simulink model "atrias_boom_nmSt_kinSw_v2"  (R2015a)
settings: Solver=ode23t  StartTime=0.0  StopTime=t_end  FixedStep=0.001  MaxStep=1e-3  RelTol=1e-3
InitFcn:
  | addpath('../common/')
  | colors
StartFcn:
  | tic
StopFcn:
  | %stopscript
values from neighbouring files (symbols this model uses):
  dt_a_dTrunk_boom = 5    [main_1_nmSt_kinSw.m]    (also in main_2_nmSt_kinSw_v2.m; main_3_nmSt_kinSw_v3.m; main_4_nmSt_kinSw_v4.m)
  dt_fade_boomCtrl = 2    [main_1_nmSt_kinSw.m]    (also in main_2_nmSt_kinSw_v2.m; main_3_nmSt_kinSw_v3.m; main_4_nmSt_kinSw_v4.m)
  initial_boom_yaw = 15*pi/180    (= 0.261799387799)    [main_2_nmSt_kinSw_v2.m]    (also in main_3_nmSt_kinSw_v3.m; main_4_nmSt_kinSw_v4.m)
  kd_boom_roll_Ctrl = 0    [main_1_nmSt_kinSw - Copy.m]    (also in main_1_nmSt_kinSw.m; main_2_nmSt_kinSw_v2.m; main_3_nmSt_kinSw_v3.m; main_4_nmSt_kinSw_v4.m)
  kd_boom_yaw_Ctrl = 0.1*kp_boom_yaw_Ctrl    (= 100000000)    [main_1_nmSt_kinSw - Copy.m]    (also in main_1_nmSt_kinSw.m = 1000000000; main_2_nmSt_kinSw_v2.m = 10000000; main_3_nmSt_kinSw_v3.m = 10000000; main_4_nmSt_kinSw_v4.m = 10000000)
  kd_motor = 0.90*2*sqrt(3.75*kp_motor)    [main_1_nmSt_kinSw - Copy.m]
  kinSw_alpha_start = 100*pi/180    (= 1.74532925199)    [main_1_nmSt_kinSw - Copy.m]    (also in main_1_nmSt_kinSw.m = 1.91986217719; main_2_nmSt_kinSw_v2.m = 1.83259571459; main_3_nmSt_kinSw_v3.m = 1.83259571459; main_4_nmSt_kinSw_v4.m = 1.83259571459)
  kinSw_alpha_tgt = 80*pi/180    (= 1.3962634016)    [main_1_nmSt_kinSw - Copy.m]    (also in main_1_nmSt_kinSw.m = 1.2217304764; main_2_nmSt_kinSw_v2.m = 1.2217304764; main_3_nmSt_kinSw_v3.m = 1.2217304764; main_4_nmSt_kinSw_v4.m = 1.2217304764)
  kinSw_t_start = 1.5    [main_1_nmSt_kinSw - Copy.m]    (also in main_1_nmSt_kinSw.m; main_2_nmSt_kinSw_v2.m = 0.5; main_3_nmSt_kinSw_v3.m = 0.5; main_4_nmSt_kinSw_v4.m = 0.5)
  kp_boom_roll_Ctrl = 0    [main_1_nmSt_kinSw - Copy.m]    (also in main_1_nmSt_kinSw.m; main_2_nmSt_kinSw_v2.m; main_3_nmSt_kinSw_v3.m; main_4_nmSt_kinSw_v4.m)
  kp_boom_yaw_Ctrl = 1e9    (= 1000000000)    [main_1_nmSt_kinSw - Copy.m]    (also in main_1_nmSt_kinSw.m = 10000000000; main_2_nmSt_kinSw_v2.m = 100000000; main_3_nmSt_kinSw_v3.m = 100000000; main_4_nmSt_kinSw_v4.m = 100000000)
  kp_motor = 3000    [main_1_nmSt_kinSw - Copy.m]
  max_back_bar_angle = 262.4*pi/180    (= 4.57974395723)    [main_1_nmSt_kinSw - Copy.m]
  max_front_bar_angle = 194.8*pi/180    (= 3.39990138288)    [main_1_nmSt_kinSw - Copy.m]
  min_back_bar_angle = 165.0*pi/180    (= 2.87979326579)    [main_1_nmSt_kinSw - Copy.m]
  min_front_bar_angle = 98.0*pi/180    (= 1.71042266695)    [main_1_nmSt_kinSw - Copy.m]
  poser_LLegAlp = (initial_l_leg_angle -pi/2)*180/pi    (= 105)    [main_2_nmSt_kinSw_v2.m]    (also in main_3_nmSt_kinSw_v3.m; main_4_nmSt_kinSw_v4.m)
  poser_LLegLen = initial_l_leg_length    (= 0.88)    [main_2_nmSt_kinSw_v2.m]    (also in main_3_nmSt_kinSw_v3.m; main_4_nmSt_kinSw_v4.m)
  poser_RLegAlp = (initial_r_leg_angle -pi/2)*180/pi    (= 75)    [main_2_nmSt_kinSw_v2.m]    (also in main_3_nmSt_kinSw_v3.m; main_4_nmSt_kinSw_v4.m)
  poser_RLegLen = initial_r_leg_length    (= 0.9)    [main_2_nmSt_kinSw_v2.m]    (also in main_3_nmSt_kinSw_v3.m; main_4_nmSt_kinSw_v4.m)
  tEnd_boomCtrl = t_end    (= 20)    [main_1_nmSt_kinSw - Copy.m]    (also in main_1_nmSt_kinSw.m = 3; main_2_nmSt_kinSw_v2.m = 7.5; main_3_nmSt_kinSw_v3.m = 7.5; main_4_nmSt_kinSw_v4.m = 7.5)
  tStart_boomCtrl = 1    [main_1_nmSt_kinSw - Copy.m]    (also in main_1_nmSt_kinSw.m = 0; main_2_nmSt_kinSw_v2.m = 0.5; main_3_nmSt_kinSw_v3.m = 0.5; main_4_nmSt_kinSw_v4.m = 0.5)
  tune_kinSw_alpha_start = kinSw_alpha_start*180/pi    (= 105)    [main_2_nmSt_kinSw_v2.m]    (also in main_3_nmSt_kinSw_v3.m; main_4_nmSt_kinSw_v4.m)
  tune_kinSw_alpha_tgt = kinSw_alpha_tgt*180/pi    (= 70)    [main_2_nmSt_kinSw_v2.m]    (also in main_3_nmSt_kinSw_v3.m; main_4_nmSt_kinSw_v4.m)
  tune_kinSw_len_min = kinSw_lclr    (= 0.7)    [main_2_nmSt_kinSw_v2.m]    (also in main_3_nmSt_kinSw_v3.m = 0.6)
  tune_kinSw_len_tgt = kinSw_len_tgt    (= 0.9)    [main_2_nmSt_kinSw_v2.m]    (also in main_3_nmSt_kinSw_v3.m)
  tune_M1_G = St_FGain_VAS*FmaxVAS    [main_2_nmSt_kinSw_v2.m]    (also in main_3_nmSt_kinSw_v3.m; main_4_nmSt_kinSw_v4.m)
  tune_M3_0 = CtrlPar_theta0*180/pi    [main_2_nmSt_kinSw_v2.m]    (also in main_3_nmSt_kinSw_v3.m; main_4_nmSt_kinSw_v4.m)
  tune_M3_D = St_GainDTh_HFL    [main_2_nmSt_kinSw_v2.m]    (also in main_3_nmSt_kinSw_v3.m; main_4_nmSt_kinSw_v4.m)
  tune_M3_P = St_GainTh_HFL    [main_2_nmSt_kinSw_v2.m]    (also in main_3_nmSt_kinSw_v3.m; main_4_nmSt_kinSw_v4.m)
  v_dTrunk_boom = 1.3    [main_1_nmSt_kinSw.m]    (also in main_2_nmSt_kinSw_v2.m; main_3_nmSt_kinSw_v3.m; main_4_nmSt_kinSw_v4.m)
undefined symbols (not defined in the file or in its folder): A1_notch_f1, A2_notch_f1, A_lpf_dtau, A_lpf_velocity, ankle_stiffness, B1_lpf_dtau, B1_lpf_velocity, B1_notch_f1, B2_lpf_dtau, B2_lpf_velocity, B2_notch_f1, b_hmotor, b_leg_spring, b_rotor, base_color_d, boom_color_d, boom_mount_to_center_diagonal, breakaway_friction, c_jointstop, contactThr, coulomb_friction, d_com, delta_phi_max, delta_phi_max_buffer, delta_phi_max_dropoff, delta_phi_min, fblink_color_d, floor_color_d, FmaxBFSH, FmaxGLU, FmaxHAM, FmaxHFL, FmaxRF, FmaxVAS, foot_color_d, FPCtrlPar, friction_linear_zone, g, gain_nodes_sea_torque, HIP_MTR_MAX_CONT_TORQUE, HIP_MTR_MAX_TORQUE, hshaft_color_d, initial_boom_pitch, initial_boom_roll, initial_hip_roll, initial_winch_angle, j_motor, k_gn, k_gt, k_leg_spring, K_notch_f1, k_phi, k_sea, Kb_leg, kd_lateral, kd_shin_max, kd_shin_min, kd_splay_max, kd_splay_min, kd_thigh_max ... (+187)
libraries: sm_lib x210, nesl_utility x140, simulink x65, simulink_extras x31, fl_lib x16, mblibv1 x2, commnoisgen2 x1
(part 4 of 16)

== system atrias_boom_nmSt_kinSw_v2/Mechanical System Layer/Right Hip Roll Joint ==
  note: Hip Roll Mechanics
  Hip Motor [Nm] : Inport
  1 / Gear Ratio : Gain  Gain=1/N_h
  Common Gear : sm_lib/Gears and Couplings/Gears/Common Gear Constraint  GearType=External  SpecificationType=PitchCircleRadii  CenterDistance=20.0  CenterDistanceUnits=cm  GearRatio=1.0  BaseGearRadius=r_hip_gearhead  BaseGearRadiusUnits=m  FollGearRadius=r_hip_shaft  FollGearRadiusUnits=m  AssemblyGearRotation=Free  BlockFunction=simmechanics.library.gears_couplings_drives.gears.common_gear
  Constant : Constant  Value=pi
  Damping : Gain  Gain=b_hmotor
  Hip Motor Frame : sm_lib/Frames and Transforms/Rigid Transform  TranslationMethod=Cartesian  TranslationLengthUnit=m  TranslationStandardAxis=+Z  TranslationStandardOffset=0  TranslationCartesianOffset=[0 r_hip_gearhead+r_hip_shaft 0]  TranslationROffset=0  TranslationROffsetUnits=m  TranslationZOffset=0  TranslationZOffsetUnits=m  TranslationThetaOffset=0  TranslationThetaOffsetUnits=deg  RotationMethod=None  RotationAngleUnits=deg  RotationStandardAxis=-Z  RotationAngle=180  RotationArbitraryAxis=[0 0 1]  FollAlignAxisA=-Z  BaseAlignAxisA=+Z  FollAlignAxisB=+Y  BaseAlignAxisB=+Y  RotationMatrix=[1 0 0; 0 1 0; 0 0 1]  BlockFunction=simmechanics.library.frames_transforms.rigid_transform
  Hip Roll Frame : sm_lib/Frames and Transforms/Rigid Transform  TranslationMethod=None  TranslationLengthUnit=m  TranslationStandardAxis=+Z  TranslationStandardOffset=0  TranslationCartesianOffset=[0 0 0]  TranslationROffset=0  TranslationROffsetUnits=m  TranslationZOffset=0  TranslationZOffsetUnits=m  TranslationThetaOffset=0  TranslationThetaOffsetUnits=deg  RotationMethod=AlignedAxes  RotationAngleUnits=deg  RotationStandardAxis=-Z  RotationAngle=180  RotationArbitraryAxis=[0 0 1]  FollAlignAxisA=+X  BaseAlignAxisA=+Z  FollAlignAxisB=+Y  BaseAlignAxisB=+Y  RotationMatrix=[1 0 0; 0 1 0; 0 0 1]  BlockFunction=simmechanics.library.frames_transforms.rigid_transform
  Hip Roll Joint : sm_lib/Joints/Revolute Joint  SenseConstraintForce=off  SenseConstraintForceX=off  SenseConstraintForceY=off  SenseConstraintForceZ=off  SenseConstraintTorque=off  SenseConstraintTorqueX=off  SenseConstraintTorqueY=off  SenseConstraintTorqueZ=off  SenseTotalForce=off  SenseTotalForceX=off  SenseTotalForceY=off  SenseTotalForceZ=off  SenseTotalTorque=off  SenseTotalTorqueX=off  SenseTotalTorqueY=off  SenseTotalTorqueZ=off  CompositeWrenchDir=FollowerOnBase  CompositeWrenchFrame=BaseFrame  EquilibriumPosition=0  EquilibriumPositionUnits=deg  SpringStiffness=0  SpringStiffnessUnits=N*m/deg  DampingCoefficient=0  DampingCoefficientUnits=N*m/(deg/s)  TorqueActuationMode=InputTorque  MotionActuationMode=ComputedMotion  SensePosition=on  SenseVelocity=on  SenseAcceleration=off  SenseTorqueForce=off  PositionTargetSpecify=on  PositionTargetPriority=High  PositionTargetValue=initial_hip_roll  PositionTargetValueUnits=rad  VelocityTargetSpecify=off  VelocityTargetPriority=High  VelocityTargetValue=0  VelocityTargetValueUnits=deg/s  BlockFunction=simmechanics.library.joints.revolute_joint
  Leg Frame : sm_lib/Frames and Transforms/Rigid Transform  TranslationMethod=None  TranslationLengthUnit=m  TranslationStandardAxis=+Z  TranslationStandardOffset=0  TranslationCartesianOffset=[0 0 0]  TranslationROffset=0  TranslationROffsetUnits=m  TranslationZOffset=0  TranslationZOffsetUnits=m  TranslationThetaOffset=0  TranslationThetaOffsetUnits=deg  RotationMethod=AlignedAxes  RotationAngleUnits=deg  RotationStandardAxis=-Z  RotationAngle=180  RotationArbitraryAxis=[0 0 1]  FollAlignAxisA=+Z  BaseAlignAxisA=+X  FollAlignAxisB=+Y  BaseAlignAxisB=+Y  RotationMatrix=[1 0 0; 0 1 0; 0 0 1]  BlockFunction=simmechanics.library.frames_transforms.rigid_transform
  "Mechanical Limits " : Subsystem
  Motor Efficiency : Gain  Gain=mu_hmotor
  Motor Joint : sm_lib/Joints/Revolute Joint  SenseConstraintForce=off  SenseConstraintForceX=off  SenseConstraintForceY=off  SenseConstraintForceZ=off  SenseConstraintTorque=off  SenseConstraintTorqueX=off  SenseConstraintTorqueY=off  SenseConstraintTorqueZ=off  SenseTotalForce=off  SenseTotalForceX=off  SenseTotalForceY=off  SenseTotalForceZ=off  SenseTotalTorque=off  SenseTotalTorqueX=off  SenseTotalTorqueY=off  SenseTotalTorqueZ=off  CompositeWrenchDir=FollowerOnBase  CompositeWrenchFrame=BaseFrame  EquilibriumPosition=0  EquilibriumPositionUnits=deg  SpringStiffness=0  SpringStiffnessUnits=N*m/deg  DampingCoefficient=0  DampingCoefficientUnits=N*m/(deg/s)  TorqueActuationMode=InputTorque  MotionActuationMode=ComputedMotion  SensePosition=off  SenseVelocity=on  SenseAcceleration=off  SenseTorqueForce=off  PositionTargetSpecify=off  PositionTargetPriority=Low  PositionTargetValue=30  PositionTargetValueUnits=deg  VelocityTargetSpecify=off  VelocityTargetPriority=High  VelocityTargetValue=0  VelocityTargetValueUnits=deg/s  BlockFunction=simmechanics.library.joints.revolute_joint
  PS-Simulink Converter : nesl_utility/PS-Simulink Converter  PhysicalDomain=network_engine_domain  SubClassName=ps_output  LeftPortType=input  RightPortType=output  PseudoPeriodic=off  Frequencies=[]  Unit=1  AffineConversion=off
  PS-Simulink Converter1 : nesl_utility/PS-Simulink Converter  PhysicalDomain=network_engine_domain  SubClassName=ps_output  LeftPortType=input  RightPortType=output  PseudoPeriodic=off  Frequencies=[]  Unit=1  AffineConversion=off
  PS-Simulink Converter3 : nesl_utility/PS-Simulink Converter  PhysicalDomain=network_engine_domain  SubClassName=ps_output  LeftPortType=input  RightPortType=output  PseudoPeriodic=off  Frequencies=[]  Unit=1  AffineConversion=off
  Rotor : sm_lib/Body Elements/Solid  InertiaType=Custom  Mass=0  MassUnits=kg  CenterOfMass=[0 0 0]  CenterOfMassUnits=m  MomentsOfInertia=i_hrotor_moments  MomentsOfInertiaUnits=kg*m^2  ProductsOfInertia=[0 0 0]  ProductsOfInertiaUnits=kg*m^2  DensityBased=on  Density=1000  DensityUnits=kg/(m^3)  GraphicType=None  MarkerShape=Sphere  MarkerSize=10  MarkerSizeUnits=m  GraphicVisPropType=AdvancedVisualProperties  GraphicDiffuseColor=hshaft_color_d  GraphicSpecularColor=[0.5 0.5 0.5 1.0]  GraphicAmbientColor=[0.15 0.15 0.15 1.0]  GraphicEmissiveColor=[0.0 0.0 0.0 1.0]  GraphicShininess=10  GraphicOpacity=1.0  GeometryShape=Cylinder  RectangleSize=[1 1]  RectangleSizeUnits=m  BrickDimensions=[1 1 1]  BrickDimensionUnits=m  CylinderRadius=0.1  CylinderRadiusUnits=m  CylinderLength=0.1  CylinderLengthUnits=m  SphereRadius=1  SphereRadiusUnits=m  EllipsoidRadii=[1 1 1]  EllipsoidRadiiUnits=m  ExtrusionCrossSection=[1 1; -1 1; -1 -1; 1 -1]  ExtrusionCrossSectionUnits=m  ExtrusionLength=1  ExtrusionLengthUnits=m  PolygonNumSides=3  PolygonOuterRadius=1  PolygonOuterRadiusUnits=m  ExtGeomFileType=STL  ExtGeomFileUnits=m  RevolutionCrossSection=[1 1; 1 -1; 2 -1; 2 1]  RevolutionCrossSectionUnits=m  RevolutionExtent=Full  RevolutionAngle=180  RevolutionAngleUnits=deg  BlockFunction=simmechanics.library.body_elements.solid
  Simulink-PS Converter : nesl_utility/Simulink-PS Converter  PhysicalDomain=network_engine_domain  SubClassName=ps_input  LeftPortType=input  RightPortType=output  PseudoPeriodic=off  Frequencies=[]  NoiseDistribution=none  NoiseParameters=[]  Unit=1  AffineConversion=off  InputFiltering=off  SimscapeFilterOrder=1  InputFilterTimeConstant=0.001  UdotUserProvided=1
  Simulink-PS Converter1 : nesl_utility/Simulink-PS Converter  PhysicalDomain=network_engine_domain  SubClassName=ps_input  LeftPortType=input  RightPortType=output  PseudoPeriodic=off  Frequencies=[]  NoiseDistribution=none  NoiseParameters=[]  Unit=1  AffineConversion=off  InputFiltering=off  SimscapeFilterOrder=1  InputFilterTimeConstant=0.001  UdotUserProvided=1
  Sum : Sum  Inputs=|+-
  Sum1 : Sum  Inputs=++|
  Torque Limiter (outside) 1 : Saturate  UpperLimit=HIP_MTR_MAX_TORQUE  LowerLimit=-HIP_MTR_MAX_TORQUE  ZeroCross=off
      settings: AttributesFormatString=Hi: %<UpperLimit>\nLo: %<LowerLimit>
  Leg Hip Conn : PMIOPort  Port=1  Side=Right
  Torso Hip Conn : PMIOPort  Port=2  Side=Left
  Hip Roll [rad] : Outport
  wires:
  Motor Efficiency/1 -> Simulink-PS Converter1/1
  Sum/1 -> Motor Efficiency/1
  Damping/1 -> Sum/2
  PS-Simulink Converter3/1 -> Damping/1
  Constant/1 -> Sum1/2
  Hip Motor [Nm]/1 -> Torque Limiter (outside) 1/1
  1 / Gear Ratio/1 -> Sum/1
  PS-Simulink Converter1/1 -> "Mechanical Limits "/1(vphi)
  Sum1/1 -> "Mechanical Limits "/2(phi)
  PS-Simulink Converter/1 -> Hip Roll [rad]/1, Sum1/1
  "Mechanical Limits "/1(tau_reaction) -> Simulink-PS Converter/1
  Torque Limiter (outside) 1/1 -> 1 / Gear Ratio/1
  connections:
  Hip Roll Frame/RConn1 -- Hip Roll Joint/LConn1 -- Hip Motor Frame/LConn1
  Simulink-PS Converter/RConn1 -- Hip Roll Joint/LConn2
  PS-Simulink Converter/LConn1 -- Hip Roll Joint/RConn2
  PS-Simulink Converter1/LConn1 -- Hip Roll Joint/RConn3
  Hip Roll Frame/LConn1 -- Torso Hip Conn/RConn1
  Leg Frame/RConn1 -- Leg Hip Conn/RConn1
  Motor Joint/RConn2 -- PS-Simulink Converter3/LConn1
  Simulink-PS Converter1/RConn1 -- Motor Joint/LConn2
  Leg Frame/LConn1 -- Common Gear/RConn1 -- Hip Roll Joint/RConn1
  Hip Motor Frame/RConn1 -- Motor Joint/LConn1
  Rotor/RConn1 -- Common Gear/LConn1 -- Motor Joint/RConn1

== system atrias_boom_nmSt_kinSw_v2/Mechanical System Layer/Torso ==
  COM Sensor : Subsystem
  COM accelerations : Scope
      settings: TimeRange=3  YMin=-750  YMax=2750  SaveName=ScopeData27
  COM dx : Scope
      settings: TimeRange=4  YMin=2.65  YMax=3.5  SaveName=ScopeData24
  COM dy : Scope
      settings: TimeRange=4  YMin=-1.25  YMax=1.5  SaveName=ScopeData32
  COM y pos : Scope
      settings: TimeRange=3  YMin=0.825  YMax=1.025  SaveName=ScopeData23
  CS1 to CS2 : sm_lib/Frames and Transforms/Rigid Transform  TranslationMethod=Cartesian  TranslationLengthUnit=m  TranslationStandardAxis=+Z  TranslationStandardOffset=0  TranslationCartesianOffset=torso_12  TranslationROffset=0  TranslationROffsetUnits=m  TranslationZOffset=0  TranslationZOffsetUnits=m  TranslationThetaOffset=0  TranslationThetaOffsetUnits=deg  RotationMethod=None  RotationAngleUnits=deg  RotationStandardAxis=+Z  RotationAngle=0  RotationArbitraryAxis=[0 0 1]  FollAlignAxisA=+X  BaseAlignAxisA=+Y  FollAlignAxisB=+Y  BaseAlignAxisB=+Z  RotationMatrix=[1 0 0; 0 1 0; 0 0 1]  BlockFunction=simmechanics.library.frames_transforms.rigid_transform
  Frame Data : Subsystem
  Hip Point to COM : sm_lib/Frames and Transforms/Rigid Transform  TranslationMethod=Cartesian  TranslationLengthUnit=m  TranslationStandardAxis=+Z  TranslationStandardOffset=0  TranslationCartesianOffset=[0 d_com 0]  TranslationROffset=0  TranslationROffsetUnits=m  TranslationZOffset=0  TranslationZOffsetUnits=m  TranslationThetaOffset=0  TranslationThetaOffsetUnits=deg  RotationMethod=None  RotationAngleUnits=deg  RotationStandardAxis=+Z  RotationAngle=0  RotationArbitraryAxis=[0 0 1]  FollAlignAxisA=+X  BaseAlignAxisA=+Y  FollAlignAxisB=+Y  BaseAlignAxisB=+Z  RotationMatrix=[1 0 0; 0 1 0; 0 0 1]  BlockFunction=simmechanics.library.frames_transforms.rigid_transform
  Mux : Mux  Inputs=2
  Solid : sm_lib/Body Elements/Solid  InertiaType=Custom  Mass=m_torso  MassUnits=kg  CenterOfMass=com_torso  CenterOfMassUnits=m  MomentsOfInertia=i_torso_moments  MomentsOfInertiaUnits=kg*m^2  ProductsOfInertia=i_torso_products  ProductsOfInertiaUnits=kg*m^2  DensityBased=on  Density=1000  DensityUnits=kg/(m^3)  GraphicType=FromGeometry  MarkerShape=Sphere  MarkerSize=10  MarkerSizeUnits=m  GraphicVisPropType=AdvancedVisualProperties  GraphicDiffuseColor=torso_color_d  GraphicSpecularColor=[0.5 0.5 0.5 1.0]  GraphicAmbientColor=[torso_color_d*0.5 1.0]  GraphicEmissiveColor=[0.0 0.0 0.0 1.0]  GraphicShininess=128  GraphicOpacity=1.0  GeometryShape=FromFile  RectangleSize=[1 1]  RectangleSizeUnits=m  BrickDimensions=[1 1 1]  BrickDimensionUnits=m  CylinderRadius=l_rad  CylinderRadiusUnits=m  CylinderLength=l_seg  CylinderLengthUnits=m  SphereRadius=1  SphereRadiusUnits=m  EllipsoidRadii=[1 1 1]  EllipsoidRadiiUnits=m  ExtrusionCrossSection=[1 1; -1 1; -1 -1; 1 -1]  ExtrusionCrossSectionUnits=m  ExtrusionLength=1  ExtrusionLengthUnits=m  PolygonNumSides=3  PolygonOuterRadius=1  PolygonOuterRadiusUnits=m  ExtGeomFileType=STL  ExtGeomFileName=../models/torso.STL  ExtGeomFileUnits=m  RevolutionCrossSection=[1 1; 1 -1; 2 -1; 2 1]  RevolutionCrossSectionUnits=m  RevolutionExtent=Full  RevolutionAngle=180  RevolutionAngleUnits=deg  BlockFunction=simmechanics.library.body_elements.solid
  Sum : Sum  Inputs=|++
  Total Energy : Scope
      settings: TimeRange=4  YMin=750  YMax=1025  SaveName=ScopeData22
  kinetic : Fcn  Expr=0.5*(u(1)^2+u(2)^2)*(m_total+m_boom/2)
  potential : Fcn  Expr=u*(m_total+m_boom/2)*g
  CS1 : PMIOPort  Port=1  Side=Right
  CS2 : PMIOPort  Port=2  Side=Left
  CS3 : PMIOPort  Port=3  Side=Left
  wires:
  COM Sensor/3(dx) -> Mux/1, COM dx/1
  COM Sensor/1(Acceleration) -> COM accelerations/1
  COM Sensor/4(dy) -> COM dy/1, Mux/2
  Mux/1 -> kinetic/1
  COM Sensor/2(y) -> COM y pos/1, potential/1
  kinetic/1 -> Sum/1
  potential/1 -> Sum/2
  Sum/1 -> Total Energy/1
  connections:
  CS1 to CS2/LConn1 -- Frame Data/LConn1 -- CS1/RConn1 -- Solid/RConn1
  CS3/RConn1 -- CS2/RConn1 -- Hip Point to COM/LConn1 -- CS1 to CS2/RConn1
  Hip Point to COM/RConn1 -- COM Sensor/LConn1

== system atrias_boom_nmSt_kinSw_v2/Mechanical System Layer/Winch ==
  note: Cable cannot push
  boom_roll_ctrl [Nm] : Inport
  Compare To Constant1 : simulink/Logic and Bit Operations/Compare To Constant  relop===  const=-1  OutDataTypeStr=boolean  ZeroCross=off
  Constant1 : Constant  Value=initial_winch_angle
  Constant2 : Constant  Value=0
  Desired Roll Velocity : Constant  Value=0
  Gain1 : Gain  Gain=kp_winch
  Gain3 : Gain  Gain=kd_winch
  PS-Simulink Converter : nesl_utility/PS-Simulink Converter  PhysicalDomain=network_engine_domain  SubClassName=ps_output  LeftPortType=input  RightPortType=output  PseudoPeriodic=off  Frequencies=[]  Unit=1  AffineConversion=off
  PS-Simulink Converter1 : nesl_utility/PS-Simulink Converter  PhysicalDomain=network_engine_domain  SubClassName=ps_output  LeftPortType=input  RightPortType=output  PseudoPeriodic=off  Frequencies=[]  Unit=1  AffineConversion=off
  Pitch Frame : sm_lib/Frames and Transforms/Rigid Transform  TranslationMethod=None  TranslationLengthUnit=m  TranslationStandardAxis=+Z  TranslationStandardOffset=0  TranslationCartesianOffset=[0 0 0]  TranslationROffset=0  TranslationROffsetUnits=m  TranslationZOffset=0  TranslationZOffsetUnits=m  TranslationThetaOffset=0  TranslationThetaOffsetUnits=deg  RotationMethod=AlignedAxes  RotationAngleUnits=rad  RotationStandardAxis=+Z  RotationAngle=0  RotationArbitraryAxis=[1 0 0]  FollAlignAxisA=-Z  BaseAlignAxisA=+X  FollAlignAxisB=+Y  BaseAlignAxisB=+Y  RotationMatrix=[1 0 0; 0 1 0; 0 0 1]  BlockFunction=simmechanics.library.frames_transforms.rigid_transform
  Roll Frame : sm_lib/Frames and Transforms/Rigid Transform  TranslationMethod=None  TranslationLengthUnit=m  TranslationStandardAxis=+Z  TranslationStandardOffset=0  TranslationCartesianOffset=[0 0 0]  TranslationROffset=0  TranslationROffsetUnits=m  TranslationZOffset=0  TranslationZOffsetUnits=m  TranslationThetaOffset=0  TranslationThetaOffsetUnits=deg  RotationMethod=AlignedAxes  RotationAngleUnits=rad  RotationStandardAxis=+Z  RotationAngle=0  RotationArbitraryAxis=[1 0 0]  FollAlignAxisA=+X  BaseAlignAxisA=-Z  FollAlignAxisB=+Y  BaseAlignAxisB=+Y  RotationMatrix=[1 0 0; 0 1 0; 0 0 1]  BlockFunction=simmechanics.library.frames_transforms.rigid_transform
  Roll Joint : sm_lib/Joints/Revolute Joint  SenseConstraintForce=off  SenseConstraintForceX=off  SenseConstraintForceY=off  SenseConstraintForceZ=off  SenseConstraintTorque=off  SenseConstraintTorqueX=off  SenseConstraintTorqueY=off  SenseConstraintTorqueZ=off  SenseTotalForce=off  SenseTotalForceX=off  SenseTotalForceY=off  SenseTotalForceZ=off  SenseTotalTorque=off  SenseTotalTorqueX=off  SenseTotalTorqueY=off  SenseTotalTorqueZ=off  CompositeWrenchDir=FollowerOnBase  CompositeWrenchFrame=BaseFrame  EquilibriumPosition=0  EquilibriumPositionUnits=deg  SpringStiffness=0  SpringStiffnessUnits=N*m/deg  DampingCoefficient=0  DampingCoefficientUnits=N*m/(deg/s)  TorqueActuationMode=InputTorque  MotionActuationMode=ComputedMotion  SensePosition=on  SenseVelocity=on  SenseAcceleration=off  SenseTorqueForce=off  PositionTargetSpecify=on  PositionTargetPriority=High  PositionTargetValue=initial_boom_roll  PositionTargetValueUnits=rad  VelocityTargetSpecify=off  VelocityTargetPriority=High  VelocityTargetValue=0  VelocityTargetValueUnits=deg/s  BlockFunction=simmechanics.library.joints.revolute_joint
  Sign1 : Signum  ZeroCross=off
  Simulink-PS Converter : nesl_utility/Simulink-PS Converter  PhysicalDomain=network_engine_domain  SubClassName=ps_input  LeftPortType=input  RightPortType=output  PseudoPeriodic=off  Frequencies=[]  NoiseDistribution=none  NoiseParameters=[]  Unit=1  AffineConversion=off  InputFiltering=off  SimscapeFilterOrder=1  InputFilterTimeConstant=0.001  UdotUserProvided=1
  Sum : Sum  Inputs=+-|
  Sum1 : Sum  Inputs=+|+
  Sum2 : Sum  Inputs=|++
  Sum3 : Sum  Inputs=+-|
  Switch : Switch  Threshold=1
  Boom : PMIOPort  Port=1  Side=Right
  Yaw Shaft : PMIOPort  Port=2  Side=Right
  Boom Roll [rad] : Outport
  wires:
  Sum/1 -> Gain1/1
  Sum1/1 -> Switch/3, Sign1/1
  Sign1/1 -> Compare To Constant1/1
  Constant2/1 -> Switch/1
  Compare To Constant1/1 -> Switch/2
  PS-Simulink Converter/1 -> Boom Roll [rad]/1, Sum/2
  PS-Simulink Converter1/1 -> Sum3/2
  Desired Roll Velocity/1 -> Sum3/1
  Sum3/1 -> Gain3/1
  Gain1/1 -> Sum1/1
  Gain3/1 -> Sum1/2
  Constant1/1 -> Sum/1
  Switch/1 -> Sum2/1
  Sum2/1 -> Simulink-PS Converter/1
  boom_roll_ctrl [Nm]/1 -> Sum2/2
  connections:
  Roll Frame/RConn1 -- Roll Joint/LConn1
  Roll Frame/LConn1 -- Yaw Shaft/RConn1
  Boom/RConn1 -- Pitch Frame/RConn1
  Pitch Frame/LConn1 -- Roll Joint/RConn1
  Roll Joint/LConn2 -- Simulink-PS Converter/RConn1
  PS-Simulink Converter/LConn1 -- Roll Joint/RConn2
  PS-Simulink Converter1/LConn1 -- Roll Joint/RConn3

== system atrias_boom_nmSt_kinSw_v2/Mechanical System Layer/Yaw Joint ==
  boom_yaw_ctrl [Nm] : Inport
  PS-Simulink Converter3 : nesl_utility/PS-Simulink Converter  PhysicalDomain=network_engine_domain  SubClassName=ps_output  LeftPortType=input  RightPortType=output  PseudoPeriodic=off  Frequencies=[]  Unit=1  AffineConversion=off
  Roll Frame : sm_lib/Frames and Transforms/Rigid Transform  TranslationMethod=None  TranslationLengthUnit=m  TranslationStandardAxis=+Z  TranslationStandardOffset=0  TranslationCartesianOffset=[0 0 0]  TranslationROffset=0  TranslationROffsetUnits=m  TranslationZOffset=0  TranslationZOffsetUnits=m  TranslationThetaOffset=0  TranslationThetaOffsetUnits=deg  RotationMethod=AlignedAxes  RotationAngleUnits=rad  RotationStandardAxis=+Z  RotationAngle=0  RotationArbitraryAxis=[1 0 0]  FollAlignAxisA=+Z  BaseAlignAxisA=+Y  FollAlignAxisB=+X  BaseAlignAxisB=+X  RotationMatrix=[1 0 0; 0 1 0; 0 0 1]  BlockFunction=simmechanics.library.frames_transforms.rigid_transform
  Simulink-PS Converter : nesl_utility/Simulink-PS Converter  PhysicalDomain=network_engine_domain  SubClassName=ps_input  LeftPortType=input  RightPortType=output  PseudoPeriodic=off  Frequencies=[]  NoiseDistribution=none  NoiseParameters=[]  Unit=1  AffineConversion=off  InputFiltering=off  SimscapeFilterOrder=1  InputFilterTimeConstant=0.001  UdotUserProvided=1
  Yaw Frame : sm_lib/Frames and Transforms/Rigid Transform  TranslationMethod=None  TranslationLengthUnit=m  TranslationStandardAxis=+Z  TranslationStandardOffset=0  TranslationCartesianOffset=[0 0 0]  TranslationROffset=0  TranslationROffsetUnits=m  TranslationZOffset=0  TranslationZOffsetUnits=m  TranslationThetaOffset=0  TranslationThetaOffsetUnits=deg  RotationMethod=AlignedAxes  RotationAngleUnits=rad  RotationStandardAxis=+Z  RotationAngle=0  RotationArbitraryAxis=[1 0 0]  FollAlignAxisA=+Y  BaseAlignAxisA=+Z  FollAlignAxisB=+X  BaseAlignAxisB=+X  RotationMatrix=[1 0 0; 0 1 0; 0 0 1]  BlockFunction=simmechanics.library.frames_transforms.rigid_transform
  Yaw Joint : sm_lib/Joints/Revolute Joint  SenseConstraintForce=off  SenseConstraintForceX=off  SenseConstraintForceY=off  SenseConstraintForceZ=off  SenseConstraintTorque=off  SenseConstraintTorqueX=off  SenseConstraintTorqueY=off  SenseConstraintTorqueZ=off  SenseTotalForce=off  SenseTotalForceX=off  SenseTotalForceY=off  SenseTotalForceZ=off  SenseTotalTorque=off  SenseTotalTorqueX=off  SenseTotalTorqueY=off  SenseTotalTorqueZ=off  CompositeWrenchDir=FollowerOnBase  CompositeWrenchFrame=BaseFrame  EquilibriumPosition=0  EquilibriumPositionUnits=deg  SpringStiffness=0  SpringStiffnessUnits=N*m/deg  DampingCoefficient=0  DampingCoefficientUnits=N*m/(deg/s)  TorqueActuationMode=InputTorque  MotionActuationMode=ComputedMotion  SensePosition=on  SenseVelocity=off  SenseAcceleration=off  SenseTorqueForce=off  PositionTargetSpecify=on  PositionTargetPriority=High  PositionTargetValue=initial_boom_yaw  PositionTargetValueUnits=rad  VelocityTargetSpecify=on  VelocityTargetPriority=High  VelocityTargetValue=initial_boom_yaw_velocity  VelocityTargetValueUnits=rad/s  BlockFunction=simmechanics.library.joints.revolute_joint
  Yaw Shaft : PMIOPort  Port=1  Side=Right
  Base : PMIOPort  Port=2  Side=Left
  Yaw [rad] : Outport
  wires:
  PS-Simulink Converter3/1 -> Yaw [rad]/1
  boom_yaw_ctrl [Nm]/1 -> Simulink-PS Converter/1
  connections:
  Yaw Frame/LConn1 -- Base/RConn1
  Yaw Joint/LConn1 -- Yaw Frame/RConn1
  Roll Frame/LConn1 -- Yaw Joint/RConn1
  Roll Frame/RConn1 -- Yaw Shaft/RConn1
  PS-Simulink Converter3/LConn1 -- Yaw Joint/RConn2
  Simulink-PS Converter/RConn1 -- Yaw Joint/LConn2

== system atrias_boom_nmSt_kinSw_v2/Mechanical System Layer/Yaw Shaft ==
  CS1 to CS2 : sm_lib/Frames and Transforms/Rigid Transform  TranslationMethod=Cartesian  TranslationLengthUnit=m  TranslationStandardAxis=+Z  TranslationStandardOffset=0  TranslationCartesianOffset=yshaft_12  TranslationROffset=0  TranslationROffsetUnits=m  TranslationZOffset=0  TranslationZOffsetUnits=m  TranslationThetaOffset=0  TranslationThetaOffsetUnits=deg  RotationMethod=None  RotationAngleUnits=deg  RotationStandardAxis=+Z  RotationAngle=0  RotationArbitraryAxis=[0 0 1]  FollAlignAxisA=+X  BaseAlignAxisA=+Y  FollAlignAxisB=+Y  BaseAlignAxisB=+Z  RotationMatrix=[1 0 0; 0 1 0; 0 0 1]  BlockFunction=simmechanics.library.frames_transforms.rigid_transform
  Frame Data : Subsystem
  Solid : sm_lib/Body Elements/Solid  InertiaType=Custom  Mass=m_yshaft  MassUnits=kg  CenterOfMass=com_yshaft  CenterOfMassUnits=m  MomentsOfInertia=i_yshaft_moments  MomentsOfInertiaUnits=kg*m^2  ProductsOfInertia=i_yshaft_products  ProductsOfInertiaUnits=kg*m^2  DensityBased=on  Density=1000  DensityUnits=kg/(m^3)  GraphicType=FromGeometry  MarkerShape=Sphere  MarkerSize=10  MarkerSizeUnits=m  GraphicVisPropType=AdvancedVisualProperties  GraphicDiffuseColor=yshaft_color_d  GraphicSpecularColor=[0.5 0.5 0.5 1.0]  GraphicAmbientColor=[yshaft_color_d*0.5 1.0]  GraphicEmissiveColor=[0.0 0.0 0.0 1.0]  GraphicShininess=128  GraphicOpacity=1.0  GeometryShape=FromFile  RectangleSize=[1 1]  RectangleSizeUnits=m  BrickDimensions=[1 1 1]  BrickDimensionUnits=m  CylinderRadius=l_rad  CylinderRadiusUnits=m  CylinderLength=l_seg  CylinderLengthUnits=m  SphereRadius=1  SphereRadiusUnits=m  EllipsoidRadii=[1 1 1]  EllipsoidRadiiUnits=m  ExtrusionCrossSection=[1 1; -1 1; -1 -1; 1 -1]  ExtrusionCrossSectionUnits=m  ExtrusionLength=1  ExtrusionLengthUnits=m  PolygonNumSides=3  PolygonOuterRadius=1  PolygonOuterRadiusUnits=m  ExtGeomFileType=STL  ExtGeomFileName=../models/boom_yaw.stl  ExtGeomFileUnits=m  RevolutionCrossSection=[1 1; 1 -1; 2 -1; 2 1]  RevolutionCrossSectionUnits=m  RevolutionExtent=Full  RevolutionAngle=180  RevolutionAngleUnits=deg  BlockFunction=simmechanics.library.body_elements.solid
  CS1 : PMIOPort  Port=1  Side=Left
  CS2 : PMIOPort  Port=2  Side=Right
  connections:
  CS2/RConn1 -- CS1 to CS2/RConn1
  CS1/RConn1 -- CS1 to CS2/LConn1 -- Solid/RConn1 -- Frame Data/LConn1

== system atrias_boom_nmSt_kinSw_v2/boom Ctrl/boom Ctrl ==
  Boom Roll [rad] : Inport
  Boom Yaw [rad] : Inport  Port=2
  Enable : EnablePort
  Constant1 : Constant  Value=initial_boom_yaw
  Constant2 : Constant  Value=l_boom+boom_mount_to_center_diagonal
  Constant3 : Constant  Value=initial_boom_roll
  Derivative : Derivative
  Derivative1 : Derivative
  Desired Roll Velocity1 : Constant  Value=0
  Desired Roll Velocity2 : Constant  Value=0
  Divide : Product  Inputs=*/
  Divide1 : Product
  Divide2 : Product
  Gain1 : Gain  Gain=kd_boom_roll_Ctrl
  Gain2 : Gain  Gain=kp_boom_roll_Ctrl
  Gain3 : Gain  Gain=kd_boom_yaw_Ctrl
  Gain4 : Gain  Gain=kp_boom_yaw_Ctrl
  Gain5 : Gain  Gain=180/pi
  Gain6 : Gain  Gain=180/pi
  Integrator1 : Integrator
  Ramp : simulink/Sources/Ramp  slope=v_dTrunk_boom/dt_a_dTrunk_boom  start=0  X0=0
  Ramp1 : simulink/Sources/Ramp  slope=-1/dt_fade_boomCtrl  start=dt_a_dTrunk_boom  X0=1
  Saturation : Saturate  UpperLimit=v_dTrunk_boom  LowerLimit=0
  Saturation1 : Saturate  UpperLimit=inf  LowerLimit=0
  Sum{1,3..4,6} (4 alike) : Sum  Inputs=+-|
  Sum2 : Sum  Inputs=+|+
  Sum5 : Sum  Inputs=+|+
  Sum7 : Sum  Inputs=++|
  boom Ctrl : Scope  NumInputPorts=4
      settings: YMin=-5~-5~-5~-5  YMax=5~5~5~5  SaveName=ScopeData10
  boom_roll_ctrl [Nm] : Outport
  boom_yaw_ctrl [Nm] : Outport  Port=2
  wires:
  Sum4/1 -> Gain2/1
  Desired Roll Velocity1/1 -> Sum6/1
  Sum6/1 -> Gain1/1
  Gain2/1 -> Sum5/1
  Gain1/1 -> Sum5/2
  Constant3/1 -> Sum4/1
  Boom Roll [rad]/1 -> Derivative/1, Sum4/2
  Derivative/1 -> Sum6/2
  Sum1/1 -> Gain4/1
  Desired Roll Velocity2/1 -> Sum3/1
  Sum3/1 -> Gain3/1
  Gain4/1 -> Sum2/1
  Gain3/1 -> Sum2/2
  Boom Yaw [rad]/1 -> Gain6/1, Derivative1/1, Sum1/2
  Derivative1/1 -> Sum3/2
  Divide/1 -> Integrator1/1
  Constant1/1 -> Sum7/1
  Sum7/1 -> Gain5/1, Sum1/1
  Integrator1/1 -> Sum7/2
  Ramp/1 -> Saturation/1
  Saturation/1 -> Divide/1
  Constant2/1 -> Divide/2
  Sum5/1 -> Divide1/1
  Divide1/1 -> boom_roll_ctrl [Nm]/1
  Sum2/1 -> Divide2/2
  Divide2/1 -> boom Ctrl/4, boom_yaw_ctrl [Nm]/1
  Ramp1/1 -> Saturation1/1
  Saturation1/1 -> boom Ctrl/3, Divide2/1, Divide1/2
  Gain5/1 -> boom Ctrl/1
  Gain6/1 -> boom Ctrl/2

== system atrias_boom_nmSt_kinSw_v2/Control/Actuator Control/Activate SEA Control ==
  SEA Control Signal [Nm] x4 : Inport
  "SEA on/off [1/0] x4 " : Inport  Port=2
  Torque Signal [Nm] x4 : Inport  Port=3
  Demux : Demux
  Demux2 : Demux
  Demux3 : Demux
  Mux6 : Mux
  Switch{,1..3} (4 alike) : Switch  Criteria=u2 ~= 0
  Torque Command [Nm] x4 : Outport
  wires:
  Demux2/2 -> Switch1/3
  Demux2/1 -> Switch/3
  Demux/1 -> Switch/1
  Switch/1 -> Mux6/1
  Switch1/1 -> Mux6/2
  Switch3/1 -> Mux6/4
  Demux3/1 -> Switch/2
  Mux6/1 -> Torque Command [Nm] x4/1
  Demux3/3 -> Switch2/2
  Demux3/2 -> Switch1/2
  Demux/3 -> Switch2/1
  Switch2/1 -> Mux6/3
  Demux/4 -> Switch3/1
  Demux2/4 -> Switch3/3
  Demux3/4 -> Switch3/2
  Demux/2 -> Switch1/1
  Demux2/3 -> Switch2/3
  SEA Control Signal [Nm] x4/1 -> Demux/1
  "SEA on/off [1/0] x4 "/1 -> Demux3/1
  Torque Signal [Nm] x4/1 -> Demux2/1

== system atrias_boom_nmSt_kinSw_v2/Control/Actuator Control/Antiresonance Compensation ==
  Torque : Inport
  Notch Filter (Flight) : DiscreteTransferFcn  Numerator=[K_notch_f1 K_notch_f1*A1_notch_f1 K_notch_f1*A2_notch_f1]  Denominator=[1 B1_notch_f1 B2_notch_f1]  SampleTime=sample_time
  Filtered Torque : Outport
  wires:
  Torque/1 -> Notch Filter (Flight)/1
  Notch Filter (Flight)/1 -> Filtered Torque/1

== system atrias_boom_nmSt_kinSw_v2/Control/Actuator Control/SEA Control Toggle ==
  enable : Inport
  tau_measured : Inport  Port=2
  tau_cmd : Inport  Port=3
  Abs : Abs
  Abs1 : Abs
  But Commanding a Small Torque? : simulink/Logic and Bit Operations/Compare To Constant  relop=<  const=sea_control_torque_cmd_small_threshold  OutDataTypeStr=boolean
  Logical Operator1 : Logic  AllPortsSameDT=off  OutDataTypeStr=boolean
  Logical Operator2 : Logic  Operator=NOT  AllPortsSameDT=off  OutDataTypeStr=boolean
  Logical Operator3 : Logic  AllPortsSameDT=off  OutDataTypeStr=boolean
  Logical Operator4 : Logic  AllPortsSameDT=off  OutDataTypeStr=boolean
  Measuring a Large Torque? (High Gains) : simulink/Logic and Bit Operations/Compare To Constant  relop=>=  const=loaded_unloaded_torque_threshold  OutDataTypeStr=boolean
  SEA Control on/off [1/0] : Outport
  wires:
  But Commanding a Small Torque?/1 -> Logical Operator1/2
  Logical Operator1/1 -> Logical Operator4/2
  tau_cmd/1 -> Abs/1
  Abs/1 -> But Commanding a Small Torque?/1
  tau_measured/1 -> Abs1/1
  Abs1/1 -> Measuring a Large Torque? (High Gains)/1
  Logical Operator3/1 -> SEA Control on/off [1/0]/1
  Logical Operator2/1 -> Logical Operator3/2
  Logical Operator4/1 -> Logical Operator2/1
  enable/1 -> Logical Operator4/1, Logical Operator3/1
  Measuring a Large Torque? (High Gains)/1 -> Logical Operator1/1

== system atrias_boom_nmSt_kinSw_v2/Control/Actuator Control/SEA Controller (Torque) ==
  phi_load [rad] x4 : Inport
  phi_gear [rad] x4 : Inport  Port=2
  tau_des sagittal [Nm] x4 : Inport  Port=3
  dtau_des sagittal [Nm] x4 : Inport  Port=4
  dphi_load [rad/s] x4 : Inport  Port=5
  dphi_gear [rad/s] x4 : Inport  Port=6
  Abs : Abs
  Antiresonance Compensation : Subsystem
  Friction Compensation : Subsystem
  Loaded Unloaded Switch : Subsystem
  P gain ramp : Lookup_n-D  NumberOfTableDimensions=1  BreakpointsForDimension1=gain_nodes_sea_torque  Table=kp_sea_torque  InternalRulePriority=Speed  RndMeth=Simplest  InputSameDT=on
  Product : Product  SampleTime=sample_time  RndMeth=Zero
  Product2 : Product  RndMeth=Zero
  Spring Stiffness : Gain  Gain=k_sea
  Spring Stiffness 1 : Gain  Gain=k_sea
  Sum1 : Sum  Inputs=-+|
  Sum10 : Sum  Inputs=|++
  Sum2 : Sum  Inputs=|+-
  Sum3 : Sum  Inputs=++|
  Sum5 : Sum  Inputs=|+-
  Sum6 : Sum  Inputs=-+|
  Sum7 : Sum  Inputs=+|+
  Torque Limiter (outside) 1 : Saturate  UpperLimit=max_sagittal_loaded_torque  LowerLimit=-max_sagittal_loaded_torque
      settings: AttributesFormatString=Hi: %<UpperLimit>\nLo: %<LowerLimit>
  Torque Limiter (outside) 3 : Saturate  UpperLimit=max_sagittal_unloaded_torque  LowerLimit=-max_sagittal_unloaded_torque
      settings: AttributesFormatString=Hi: %<UpperLimit>\nLo: %<LowerLimit>
  Torque Threshold : simulink/Logic and Bit Operations/Compare To Constant  relop=>=  const=loaded_unloaded_torque_threshold  OutDataTypeStr=boolean
  critical damping : Subsystem
  tau_cmd sagittal [Nm] x4 : Outport
  tau_measured [Nm] x4 : Outport  Port=2
  wires:
  Product2/1 -> Sum7/2
  Sum2/1 -> Product2/2
  Sum5/1 -> Product/2
  dphi_gear [rad/s] x4/1 -> Friction Compensation/1(Motor Velocity [rad/s]), Sum6/2
  dphi_load [rad/s] x4/1 -> Sum6/1
  Spring Stiffness 1/1 -> Sum2/2
  Sum6/1 -> Spring Stiffness 1/1
  dtau_des sagittal [Nm] x4/1 -> Sum2/1
  tau_des sagittal [Nm] x4/1 -> Sum5/1
  phi_gear [rad] x4/1 -> Sum1/2
  phi_load [rad] x4/1 -> Sum1/1
  Sum1/1 -> Spring Stiffness/1
  Spring Stiffness/1 -> Sum3/1, Sum5/2, Abs/1, tau_measured [Nm] x4/1
  Sum10/1 -> Antiresonance Compensation/1(Torque), Torque Limiter (outside) 1/1
  P gain ramp/1 -> critical damping/1(p gain), Product/1
  Product/1 -> Sum7/1
  Sum7/1 -> Sum3/2
  Torque Limiter (outside) 1/1 -> Loaded Unloaded Switch/1(Loaded Signal)
  Torque Limiter (outside) 3/1 -> Loaded Unloaded Switch/2(Unloaded Signal)
  Antiresonance Compensation/1(Filtered Torque) -> Torque Limiter (outside) 3/1
  Friction Compensation/1(Friction Compensation [Nm]) -> Sum10/2
  Loaded Unloaded Switch/1(Signal) -> tau_cmd sagittal [Nm] x4/1
  Torque Threshold/1 -> Loaded Unloaded Switch/3(Loaded/Unloaded [1/0] x4)
  Abs/1 -> P gain ramp/1, Torque Threshold/1
  Sum3/1 -> Sum10/1
  critical damping/1(d gain) -> Product2/1

== system atrias_boom_nmSt_kinSw_v2/Control/Behavior Control/Add Limit Avoidance PD Torques ==
  tau_des [Nm] x6 : Inport
  Mux4 : Mux  Inputs=2
  Selector2 : Selector  InputPortWidth=6  Indices=[1 2 4 5]
  Selector3 : Selector  InputPortWidth=6  Indices=[3 6]
  Selector8 : Selector  InputPortWidth=6  Indices=[1 2 5 3 4 6]
  Zero-Order Hold (1kHz)4 : ZeroOrderHold  SampleTime=sample_time
  mechanical limit avoidance : Subsystem
  tau_des w/PD [Nm] x6 : Outport
  wires:
  Zero-Order Hold (1kHz)4/1 -> Selector2/1, Selector3/1
  tau_des [Nm] x6/1 -> Zero-Order Hold (1kHz)4/1
  Selector8/1 -> tau_des w/PD [Nm] x6/1
  Mux4/1 -> Selector8/1
  Selector3/1 -> Mux4/2
  Selector2/1 -> mechanical limit avoidance/1(tau_des [Nm]x4)
  mechanical limit avoidance/1(tau_des + pd [Nm]x4) -> Mux4/1

== system atrias_boom_nmSt_kinSw_v2/Control/Behavior Control/Lateral Motor Control ==
  note: PD + Buckling Compensation
  Lateral Control1 : MATLAB Function  TreatAsAtomicUnit=on
  Left Lateral Torque Saturation : Saturate  UpperLimit=max_torque_lateral  LowerLimit=-max_torque_lateral
      settings: AttributesFormatString=Top: %<UpperLimit>\nBottom: %<LowerLimit>
  Right Lateral Torque Saturation : Saturate  UpperLimit=max_torque_lateral  LowerLimit=-max_torque_lateral
      settings: AttributesFormatString=Top: %<UpperLimit>\nBottom: %<LowerLimit>
  percent body weight : Gain  Gain=(m_total*g)
  percent body weight1 : Gain  Gain=(m_total*g)
  tau_lateral_R : Outport
  tau_lateral_L : Outport  Port=2
  wires:
  Lateral Control1/1(tau_r) -> Right Lateral Torque Saturation/1
  Lateral Control1/2(tau_l) -> Left Lateral Torque Saturation/1
  Right Lateral Torque Saturation/1 -> tau_lateral_R/1
  Left Lateral Torque Saturation/1 -> tau_lateral_L/1
  [Rphi_Lat] -> Lateral Control1/1(qLateralR)
  [Rdphi_Lat] -> Lateral Control1/2(dqLateralR)
  [Lphi_Lat] -> Lateral Control1/3(qLateralL)
  [Ldphi_Lat] -> Lateral Control1/4(dqLateralL)
  [RLLoad] -> percent body weight/1
  [LLLoad] -> percent body weight1/1
  percent body weight/1 -> Lateral Control1/5(F_leg_R)
  percent body weight1/1 -> Lateral Control1/6(F_leg_L)

== system atrias_boom_nmSt_kinSw_v2/Control/Behavior Control/Monitors ==
  Gain{,1..8} (9 alike) : Gain  Gain=180/pi
  NM LStim : Scope  NumInputPorts=6
      settings: YMin=-5~-5~-5~-5~-5~-5  YMax=5~5~5~5~5~5  SaveName=ScopeData4
  NM RStim : Scope  NumInputPorts=6
      settings: YMin=-5~-5~-5~-5~-5~-5  YMax=5~5~5~5~5~5  SaveName=ScopeData3
  robot angles : Scope  NumInputPorts=4
      settings: YMin=-5~-5~-5~-5  YMax=5~5~5~5  SaveName=ScopeData7
  robot torque : Scope  NumInputPorts=6
      settings: YMin=-5~-5~-5~-5~-5~-5  YMax=5~5~5~5~5~5  SaveName=ScopeData9
  torso : Scope  NumInputPorts=3
      settings: YMin=-5~-5~-5  YMax=5~5~5  SaveName=ScopeData8
  virtual angles : Scope  NumInputPorts=5
      settings: YMin=-5~-5~-5~-5~-5  YMax=5~5~5~5~5  SaveName=ScopeData6
  virtual torque : Scope  NumInputPorts=6
      settings: YMin=-5~-5~-5~-5~-5~-5  YMax=5~5~5~5~5~5  SaveName=ScopeData2
  wires:
  [Rphi_thigh] -> Gain2/1
  [Rphi_shin] -> Gain3/1
  [Lphi_thigh] -> Gain4/1
  [Lphi_shin] -> Gain5/1
  Gain2/1 -> robot angles/1  "Rthigh"
  Gain3/1 -> robot angles/2  "Rshin"
  Gain4/1 -> robot angles/3  "Lthigh"
  Gain5/1 -> robot angles/4  "Lshin"
  Gain8/1 -> virtual angles/5  "Lknee"
  Gain1/1 -> virtual angles/2  "Rhip"
  [theta] -> Gain/1
  [Rphi12] -> Gain6/1
  [Lphi23] -> Gain7/1
  Gain6/1 -> virtual angles/3  "Rknee"
  Gain7/1 -> virtual angles/4  "Lhip"
  [Lphi12] -> Gain8/1
  Gain/1 -> virtual angles/1  "theta"
  [Rphi23] -> Gain1/1
  [Rshin_ctrl_trq] -> robot torque/1  "Rshin"
  [Rthigh_ctrl_trq] -> robot torque/2  "Rthigh"
  [RLat_ctrl_trq] -> robot torque/3  "RLat"
  [Lshin_ctrl_trq] -> robot torque/4  "Lshin"
  [Lthigh_ctrl_trq] -> robot torque/5  "Lthigh"
  [LLat_ctrl_trq] -> robot torque/6  "LLat"
  [LM12] -> virtual torque/3  "Lknee"
  [LM23] -> virtual torque/4  "Lhip"
  [RM23] -> virtual torque/2  "Rhip"
  [RM12] -> virtual torque/1  "Rknee"
  [LLLoad] -> virtual torque/6  "LLoad"
  [RLLoad] -> virtual torque/5  "RLoad"
  [LStimHFL] -> NM LStim/1  "HFL"
  [LStimGLU] -> NM LStim/2  "GLU"
  [LStimHAM] -> NM LStim/3  "HAM"
  [LStimRF] -> NM LStim/4  "RF"
  [LStimVAS] -> NM LStim/5  "VAS"
  [LStimBFSH] -> NM LStim/6  "BFSH"
  [RStimHFL] -> NM RStim/1  "HFL"
  [RStimGLU] -> NM RStim/2  "GLU"
  [RStimHAM] -> NM RStim/3  "HAM"
  [RStimRF] -> NM RStim/4  "RF"
  [RStimVAS] -> NM RStim/5  "VAS"
  [RStimBFSH] -> NM RStim/6  "BFSH"
  [xTorso] -> torso/1  "x"
  [yOffTorso] -> torso/2  "yOff"
  [dxTorso] -> torso/3  "dx"
